simulink model "funcion_transferencia"  (R2020b)
settings: Solver=VariableStepAuto  StartTime=0.0  StopTime=2  RelTol=1e-3
undefined symbols (not defined in the file): B, J, K, La, Ra
settings Model: Creator=petir  LastModifiedBy=petir

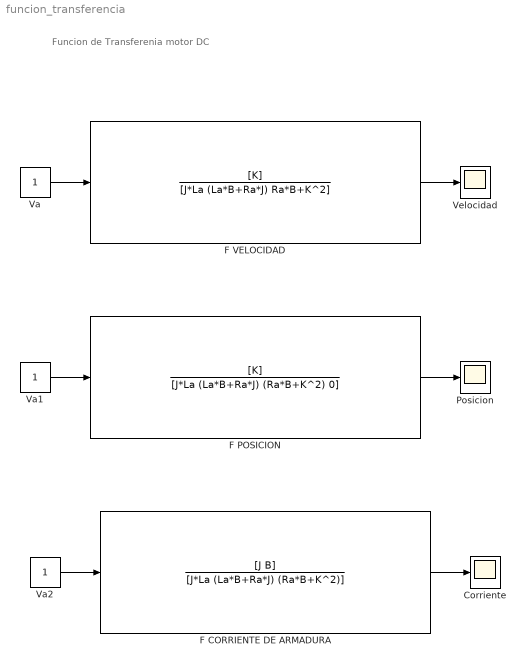
== system funcion_transferencia ==
  note: Funcion de Transferenia motor DC
  Corriente : Scope
  F CORRIENTE DE ARMADURA : TransferFcn  Numerator=[J B]  Denominator=[J*La (La*B+Ra*J) (Ra*B+K^2)]
  F POSICION : TransferFcn  Numerator=[K]  Denominator=[J*La (La*B+Ra*J) (Ra*B+K^2) 0]
  F VELOCIDAD : TransferFcn  Numerator=[K]  Denominator=[J*La (La*B+Ra*J) Ra*B+K^2]
  Posicion : Scope
  Va : Constant
  Va1 : Constant
  Va2 : Constant
  Velocidad : Scope
  wires:
  F VELOCIDAD/1 -> Velocidad/1
  Va/1 -> F VELOCIDAD/1
  Va1/1 -> F POSICION/1
  F POSICION/1 -> Posicion/1
  F CORRIENTE DE ARMADURA/1 -> Corriente/1
  Va2/1 -> F CORRIENTE DE ARMADURA/1
